simulink model "WhiteBlancing_using_Intensity_Values_of_Background"  (R2016a)
settings: Solver=VariableStepAuto  StartTime=0.0  StopTime=inf  RelTol=1e-3
undefined symbols (not defined in the file): none, Rec, SDTV, videoinput
libraries: visionconversions x2, imaqlib x1, visionsinks x1
settings Model: Creator=YASARA  LastModifiedBy=YASARA

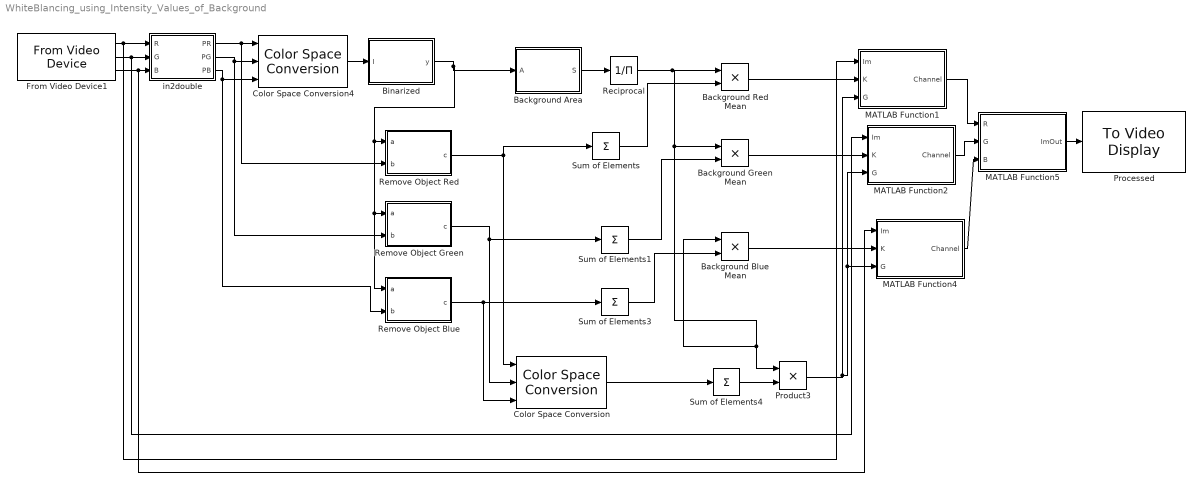
== system WhiteBlancing_using_Intensity_Values_of_Background ==
  Background Area : MATLAB Function  TreatAsAtomicUnit=on
  Background Blue Mean : Product  OutDataTypeStr=uint8
  Background Green Mean : Product  OutDataTypeStr=uint8
  Background Red Mean : Product  OutDataTypeStr=uint8
  Binarized : MATLAB Function  TreatAsAtomicUnit=on
  Color Space Conversion : visionconversions/Color Space  Conversion  conversion=Obsolete  conversionActive=R'G'B' to intensity  wp_str=D65  rec=Rec. 601 (SDTV)  sys=1125/60/2:1  imagePorts=Separate color signals
  Color Space Conversion4 : visionconversions/Color Space  Conversion  conversion=Obsolete  conversionActive=R'G'B' to intensity  wp_str=D65  rec=Rec. 601 (SDTV)  sys=1125/60/2:1  imagePorts=Separate color signals
  From Video Device1 : imaqlib/From Video Device  DeviceMenu=winvideo 1 (Integrated Webcam)  Device=winvideo 1 (Integrated Webcam)  ObjConstructor=videoinput('winvideo', 1)  VideoFormatMenu=YUY2_160x120  VideoFormat=YUY2_160x120  VideoSource=input1  ROIPosition=[0 0 120 160]  EnableHWTrigger=off  TriggerConfiguration=none/none  SampleTime=1/30  OutputPortsMode=Separate color signals  DataType=uint8  CanDoHWTrigger=no  ReturnedColorSpace=rgb  BlockHandle=44.0042  ROIWidth=160  ROIHeight=120  ROIColumn=0  ROIRow=0  EngXMLPath=C:\Program Files\MATLAB\R2016a\toolbox\imaq\imaq\private  DevXMLPath=C:\MATLAB\SupportPackages\R2016a\toolbox\imaq\supportpackages\genericvideo\adaptor\win64  EngLibPath=C:\Program Files\MATLAB\R2016a\toolbox\imaq\imaqblks\imaqmex\win64  ColorSpace=rgb  BayerSensorAlignment=grbg
  MATLAB Function1 : MATLAB Function  TreatAsAtomicUnit=on
  MATLAB Function2 : MATLAB Function  TreatAsAtomicUnit=on
  MATLAB Function4 : MATLAB Function  TreatAsAtomicUnit=on
  MATLAB Function5 : MATLAB Function  TreatAsAtomicUnit=on
  Processed : visionsinks/To Video Display  windowSizeMode=Normal  openAtMdlStart=on  fullScreen=off  videoWindowX=252  videoWindowY=213  saveWindowSize=off  videoWindowWidth=512  videoWindowHeight=384  inputColorFormat=RGB  inputType=Obsolete  imagePorts=One multidimensional signal  OutputDevice=On-screen video monitor  dataOrg=Column-major  isWindowOpen=off
  Product3 : Product  OutDataTypeStr=uint8
  Reciprocal : Product  Inputs=/  OutDataTypeStr=double  SaturateOnIntegerOverflow=on  RndMeth=Zero
  Remove Object Blue : MATLAB Function  TreatAsAtomicUnit=on
  Remove Object Green : MATLAB Function  TreatAsAtomicUnit=on
  Remove Object Red : MATLAB Function  TreatAsAtomicUnit=on
  Sum of Elements{,1,3..4} (4 alike) : Sum  Inputs=+
  in2double : MATLAB Function  TreatAsAtomicUnit=on
  wires:
  Color Space Conversion4/1 -> Binarized/1(I)
  Remove Object Red/1(c) -> Sum of Elements/1, Color Space Conversion/1
  Remove Object Green/1(c) -> Sum of Elements1/1, Color Space Conversion/2
  Remove Object Blue/1(c) -> Sum of Elements3/1, Color Space Conversion/3
  Reciprocal/1 -> Background Green Mean/1, Product3/1, Background Blue Mean/1, Background Red Mean/1
  Binarized/1(y) -> Background Area/1(A), Remove Object Blue/1(a), Remove Object Green/1(a), Remove Object Red/1(a)
  in2double/1(PR) -> Remove Object Red/2(b), Color Space Conversion4/1
  in2double/2(PG) -> Remove Object Green/2(b), Color Space Conversion4/2
  in2double/3(PB) -> Remove Object Blue/2(b), Color Space Conversion4/3
  Background Red Mean/1 -> MATLAB Function1/2(K)
  Background Green Mean/1 -> MATLAB Function2/2(K)
  Background Blue Mean/1 -> MATLAB Function4/2(K)
  Color Space Conversion/1 -> Sum of Elements4/1
  Sum of Elements/1 -> Background Red Mean/2
  Product3/1 -> MATLAB Function1/3(G), MATLAB Function2/3(G), MATLAB Function4/3(G)
  Sum of Elements1/1 -> Background Green Mean/2
  Sum of Elements3/1 -> Background Blue Mean/2
  Sum of Elements4/1 -> Product3/2
  Background Area/1(S) -> Reciprocal/1
  MATLAB Function2/1(Channel) -> MATLAB Function5/2(G)
  MATLAB Function4/1(Channel) -> MATLAB Function5/3(B)
  MATLAB Function5/1(ImOut) -> Processed/1
  MATLAB Function1/1(Channel) -> MATLAB Function5/1(R)
  From Video Device1/1 -> MATLAB Function1/1(Im), in2double/1(R)
  From Video Device1/2 -> MATLAB Function2/1(Im), in2double/2(G)
  From Video Device1/3 -> MATLAB Function4/1(Im), in2double/3(B)

== matlab function WhiteBlancing_using_Intensity_Values_of_Background/MATLAB Function1 ==
  data: Im input; K input; Channel output; G input
function Channel = fcn(Im,K,G)
Channel = uint8(double(Im) *double(G)/double(K));
return

== matlab function WhiteBlancing_using_Intensity_Values_of_Background/MATLAB Function2 ==
  data: Im input; K input; Channel output; G input
function Channel = fcn(Im,K,G)
Channel = uint8(double(Im) *double(G)/double(K));
return

== matlab function WhiteBlancing_using_Intensity_Values_of_Background/Background Area ==
  data: A input; S output
function S = fcn(A)
%#codegen
S = sum(A(:))/100;

== matlab function WhiteBlancing_using_Intensity_Values_of_Background/MATLAB Function4 ==
  data: Im input; K input; Channel output; G input
function Channel = fcn(Im,K,G)
Channel = uint8(double(Im) *double(G)/double(K));
return

== matlab function WhiteBlancing_using_Intensity_Values_of_Background/MATLAB Function5 ==
  data: R input; G input; B input; ImOut output
function ImOut = fcn(R,G,B)
ImOut = cat(3, R, G, B);
return

== matlab function WhiteBlancing_using_Intensity_Values_of_Background/in2double ==
  data: R input; G input; PR output; B input; PG output; PB output
function [PR,PG,PB] = fcn(R,G,B)
%#codegen
Im=cat(3,R,G,B);
PR= im2double(R);
PG= im2double(G);
PB= im2double(B);
return

== matlab function WhiteBlancing_using_Intensity_Values_of_Background/Remove Object Green ==
  data: a input; b input; c output
function c = fcn(a,b)
%#codegen
c=a.*b;
return

== matlab function WhiteBlancing_using_Intensity_Values_of_Background/Binarized ==
  data: I input; y output
function y = fcn(I)
%#codegen
y=logical(I);
coder.extrinsic('graythresh');
level = graythresh(I);
BW = im2bw(I,level);

== matlab function WhiteBlancing_using_Intensity_Values_of_Background/Remove Object Blue ==
  data: a input; b input; c output
function c = fcn(a,b)
%#codegen
c=a.*b;
return

== matlab function WhiteBlancing_using_Intensity_Values_of_Background/Remove Object Red ==
  data: a input; b input; c output
function c = fcn(a,b)
%#codegen
c=a.*b;
return
